simulink model "diagram_digital_vector"  (Simulink 7.5)
settings: Solver=ode4  StartTime=0.0  StopTime=10.0  FixedStep=0.001  RelTol=1e-3
PreLoadFcn:
  | diagram_digital_vector_param
values from neighbouring files (symbols this model uses):
  A = [ 0  1  0;       0  0  1;      -3 -7 -5]    [diagram_digital_vector_param.m]
  B = [1;  -2;  5]    [diagram_digital_vector_param.m]
  C = [1  0  0]    [diagram_digital_vector_param.m]
  x0 = [0; 0; 0]    [diagram_digital_vector_param.m]
settings Model: Creator=Dell  LastModifiedBy=Dell

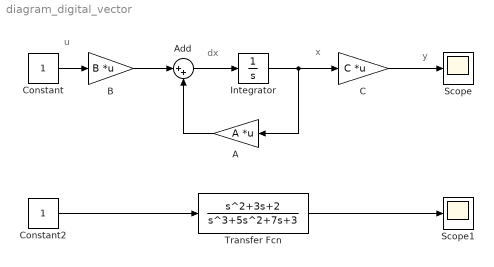
== system diagram_digital_vector ==
  note: x
  note: dx
  note: u
  note: y
  A : Gain  Gain=A  Multiplication=Matrix(K*u)  ParameterDataType=fixdt(1, 16)  ParameterScaling=2^0  OutDataType=fixdt(1, 16)  OutScaling=2^0
  Add : Sum  Inputs=|++  OutDataType=fixdt(1, 16)  OutScaling=2^-10
  B : Gain  Gain=B  Multiplication=Matrix(K*u)  ParameterDataType=fixdt(1, 16)  ParameterScaling=2^0  OutDataType=fixdt(1, 16)  OutScaling=2^0
  C : Gain  Gain=C  Multiplication=Matrix(K*u)  ParameterDataType=fixdt(1, 16)  ParameterScaling=2^0  OutDataType=fixdt(1, 16)  OutScaling=2^0
  Constant : Constant  OutDataType=fixdt(1, 16)  OutScaling=2^0
  Constant2 : Constant  OutDataType=fixdt(1, 16)  OutScaling=2^0
  Integrator : Integrator  InitialCondition=x0
  Scope : Scope
      settings: TimeRange=10  YMin=0  YMax=1  MaxDataPoints=10000
  Scope1 : Scope
      settings: TimeRange=10  YMin=0  YMax=1  SaveName=ScopeData2  MaxDataPoints=10000
  Transfer Fcn : TransferFcn  Numerator="[1 3  2]"  Denominator="[1 5  7 3]"
  wires:
  Integrator/1 -> A/1, C/1
  Add/1 -> Integrator/1
  A/1 -> Add/2
  B/1 -> Add/1
  Constant/1 -> B/1
  C/1 -> Scope/1
  Constant2/1 -> Transfer Fcn/1
  Transfer Fcn/1 -> Scope1/1
